simulink model "sim1"  (R2017b)
settings: Solver=VariableStepAuto  StartTime=0.0  StopTime=10.0  RelTol=1e-3
settings Model: Creator=Administrator  LastModifiedBy=Administrator

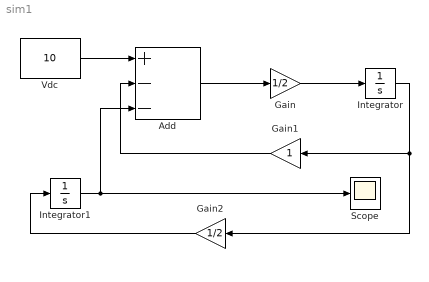
== system sim1 ==
  Add : Sum  Inputs=+--
  Gain : Gain  Gain=1/2
  Gain1 : Gain
  Gain2 : Gain  Gain=1/2
  Integrator : Integrator
  Integrator1 : Integrator
  Scope : Scope
  "Vdc " : Constant  Value=10
  wires:
  "Vdc "/1 -> Add/1
  Add/1 -> Gain/1
  Gain/1 -> Integrator/1
  Integrator/1 -> Gain2/1, Gain1/1
  Gain1/1 -> Add/2
  Gain2/1 -> Integrator1/1
  Integrator1/1 -> Scope/1, Add/3
